simulink model "AC_base_1_VSM_2_22a"  (R2022a)
settings: Solver=ode3  StartTime=0.0  StopTime=8  FixedStep=HWSampleTime  RelTol=1e-3
undefined symbols (not defined in the file): ControlSampleTime, DiscIntNeverNeededParam, HWSampleTime, Ipwm_back, Ipwm_off, LCL, Manage, Oversample, Param, scaling_factor, SM, Ts, V_DC, VSMCTRL
libraries: fl_lib x100, nesl_utility x63, simulink x38, FriedrichLibrary x38, ee_lib x20, simulink_extras x14, TriphaseHardwaremodule x12, spsEdgeDetectorLib x2, StateMachines x2, slpidlib x2, spsPower3phInstantaneousLib x1
(part 2 of 7)

== system AC_base_1_VSM_2_22a/Variant Subsystem3/VSM/Inverter AverageMdl LC SimScape2/Modul F30 fixed DC voltage Average SimScape ==
  ctrl : Inport
  Bus Selector : BusSelector  OutputSignals=connect
  Phase Splitter : ee_lib/Connectors & References/Phase Splitter
  Rate Transition1 : RateTransition  Commented=on  Integrity=off  InitialCondition=-1  OutPortSampleTime=ControlSampleTime
  S_connect : ee_lib/Switches & Breakers/SPST Switch (Three-Phase)  R_closed=1e-9 Ohm  G_open=1e-6 1/Ohm  threshold=0.5 V  i_vT_specify=off  i_vT_priority=None  i_vT=0 A  i_vT_nominal_specify=off  i_vT_nominal_value=1  i_vT_nominal_unit=A  I_specify=off  I_priority=None  I=[ 0 0 0 ] A  I_nominal_specify=off  I_nominal_value=1  I_nominal_unit=A  V_specify=off  V_priority=None  V=[ 0 0 0 ] V  V_nominal_specify=off  V_nominal_value=1  V_nominal_unit=V  i_a_specify=off  i_a_priority=None  i_a=0 A  i_a_nominal_specify=off  i_a_nominal_value=1  i_a_nominal_unit=A  v_a_specify=off  v_a_priority=None  v_a=0 V  v_a_nominal_specify=off  v_a_nominal_value=1  v_a_nominal_unit=V  i_b_specify=off  i_b_priority=None  i_b=0 A  i_b_nominal_specify=off  i_b_nominal_value=1  i_b_nominal_unit=A  v_b_specify=off  v_b_priority=None  v_b=0 V  v_b_nominal_specify=off  v_b_nominal_value=1  v_b_nominal_unit=V  i_c_specify=off  i_c_priority=None  i_c=0 A  i_c_nominal_specify=off  i_c_nominal_value=1  i_c_nominal_unit=A  v_c_specify=off  v_c_priority=None  v_c=0 V  v_c_nominal_specify=off  v_c_nominal_value=1  v_c_nominal_unit=V
      settings: InternalSimscapePortConfiguration="{\"Bottom\":[],\"Left\":[{\"id\":\"vT\",\"label\":\"vT\",\"type\":\"input\"},{\"id\":\"N1\",\"label\":\"~1\",\"type\":\"foundation.electrical.three_phase\"}],\"Right\":[{\"id\":\"N2\",\"label\":\"~2\",\"type\":\"foundation.electrical.three_phase\"}],\"Top\":[]}"
  Simulink-PS Converter : nesl_utility/Simulink-PS Converter  PhysicalDomain=network_engine_domain  SubClassName=ps_input  LeftPortType=input  RightPortType=output  PseudoPeriodic=off  Frequencies=[]  NoiseDistribution=none  NoiseParameters=[]  Unit=1  AffineConversion=off  FilteringAndDerivatives=zero  SimscapeFilterOrder=1  InputFilterTimeConstant=0.001  UdotUserProvided=1
  ctrlSelect3 : Subsystem
  measMerge3 : Subsystem
  simscape_bridgefilter_aca : Subsystem  mask{L1=L1, R_L1=R_L1, C1=C1, R_C1=R_C1}
      mask prompts: L1 "Inductance L1 [H]"; R_L1 "Resistance of L1 [Ohm]"; C1 "Capacitance C1 [F]"; R_C1 "Parallel resistance of C1 [Ohm]"
      mask DialogControl LC Prompt: LC(L)(C)
      mask DialogControl GrpLC Prompt: LC(L)(C)-Filter
  simscape_bridgefilter_aca1 : Subsystem  mask{L1=L1, R_L1=R_L1, C1=C1, R_C1=R_C1}
      mask prompts: L1 "Inductance L1 [H]"; R_L1 "Resistance of L1 [Ohm]"; C1 "Capacitance C1 [F]"; R_C1 "Parallel resistance of C1 [Ohm]"
      mask DialogControl LC Prompt: LC(L)(C)
      mask DialogControl GrpLC Prompt: LC(L)(C)-Filter
  simscape_bridgefilter_aca2 : Subsystem  mask{L1=L1, R_L1=R_L1, C1=C1, R_C1=R_C1}
      mask prompts: L1 "Inductance L1 [H]"; R_L1 "Resistance of L1 [Ohm]"; C1 "Capacitance C1 [F]"; R_C1 "Parallel resistance of C1 [Ohm]"
      mask DialogControl LC Prompt: LC(L)(C)
      mask DialogControl GrpLC Prompt: LC(L)(C)-Filter
  N : PMIOPort  Side=Left
  ABC : PMIOPort  Port=2  Side=Right
  meas : Outport  VectorParamsAs1DForOutWhenUnconnected=off
  measf : Outport  Port=2  VectorParamsAs1DForOutWhenUnconnected=off
  wires:
  ctrlSelect3/1(ctrl1) -> Bus Selector/1, simscape_bridgefilter_aca/1(ctrl)
  [ctrl3] -> simscape_bridgefilter_aca2/1(ctrl)
  [ctrl2] -> simscape_bridgefilter_aca1/1(ctrl)
  ctrlSelect3/2(ctrl2) -> [ctrl2]
  ctrlSelect3/3(ctrl3) -> [ctrl3]
  ctrl/1 -> ctrlSelect3/1(ctrl)
  [meas2] -> measMerge3/2(meas2)
  simscape_bridgefilter_aca2/1(meas) -> [meas3]
  simscape_bridgefilter_aca1/1(meas) -> [meas2]
  [meas3] -> measMerge3/3(meas3)
  simscape_bridgefilter_aca/1(meas) -> measMerge3/1(meas1)
  measMerge3/1(meas) -> meas/1, measf/1
  Bus Selector/1 -> [connect]  "<connect>"
  [connect] -> Simulink-PS Converter/1
  connections:
  simscape_bridgefilter_aca/LConn2 -- simscape_bridgefilter_aca1/LConn2 -- simscape_bridgefilter_aca2/LConn2 -- N/RConn1
  simscape_bridgefilter_aca/RConn1 -- simscape_bridgefilter_aca2/RConn1 -- simscape_bridgefilter_aca1/RConn1
  simscape_bridgefilter_aca2/LConn1 -- Phase Splitter/RConn3
  Phase Splitter/RConn1 -- simscape_bridgefilter_aca/LConn1
  simscape_bridgefilter_aca1/LConn1 -- Phase Splitter/RConn2
  Simulink-PS Converter/RConn1 -- S_connect/LConn1
  S_connect/LConn2 -- ABC/RConn1
  S_connect/RConn1 -- Phase Splitter/LConn1

== system AC_base_1_VSM_2_22a/Variant Subsystem3/VSM/VSM1/MeasInv1 ==
  SimOut : Inport
  Bus Selector1 : BusSelector  OutputSignals=meas_u_dc,meas_u_cap,meas_u_out,meas_i_inverter,meas_i_out,connection_state,enabled
  Meas_Inv1 : Scope  NumInputPorts=7
  To Workspace1 : ToWorkspace  VariableName=MeasAC_Ucap  SampleTime=-1
  To Workspace2 : ToWorkspace  VariableName=MeasAC_Uout  SampleTime=-1
  To Workspace3 : ToWorkspace  VariableName=MeasAC_Iinv  SampleTime=-1
  To Workspace4 : ToWorkspace  VariableName=MeasAC_Iout  SampleTime=-1
  To Workspace7 : ToWorkspace  VariableName=MeasAC_Udc  SampleTime=-1
  wires:
  Bus Selector1/7 -> Meas_Inv1/7  "<enabled>"
  Bus Selector1/6 -> Meas_Inv1/6  "<connection_state>"
  Bus Selector1/5 -> To Workspace4/1, Meas_Inv1/5  "<meas_i_out>"
  Bus Selector1/4 -> To Workspace3/1, Meas_Inv1/4  "<meas_i_inverter>"
  Bus Selector1/3 -> To Workspace2/1, Meas_Inv1/3  "<meas_u_out>"
  Bus Selector1/2 -> To Workspace1/1, Meas_Inv1/2  "<meas_u_cap>"
  Bus Selector1/1 -> To Workspace7/1, Meas_Inv1/1  "<meas_u_dc>"
  SimOut/1 -> Bus Selector1/1

== system AC_base_1_VSM_2_22a/Variant Subsystem3/VSM/VSM1/VSM ==
  cmd : Inport
  meas : Inport  Port=2
  BUS_GENERATION : Subsystem
  CONTROL : Subsystem
  MANAGEMENT : Subsystem  mask(VSMCC Management){Mgn=Ctrl.Mgn}
      mask prompts: Mgn "Mgn Parameters"
      mask help:
      | Mgn(.PQSpRateUp, .PQSpRateDown, PQSpMax, .PQSpMin)
      |
      | Parameter nicht auf der Maske:
      | ControlSampleTime
  Meas : Subsystem  mask(Messeinrichtung für VSM mit CC){PU=pu, PLL=Ctrl.PLL}
      mask prompts: PU "PU System"; PLL "PLL Parameters"
      mask help:
      | PU System(.Vb, .Ib)
      |
      | PLL Parameter (.kp, .ki)
      |
      | Parameter nicht auf der Maske:
      | NrChannels
      | ControlSampleTime
  ctrl : Outport  VectorParamsAs1DForOutWhenUnconnected=off  LockScale=on
  feedback : Outport  Port=2  VectorParamsAs1DForOutWhenUnconnected=off
  diag : Outport  Port=3  VectorParamsAs1DForOutWhenUnconnected=off
  wires:
  meas/1 -> Meas/1(MEASIN)
  cmd/1 -> MANAGEMENT/1(CMD)
  CONTROL/1(CONTROL) -> Meas/2("CONTROL "), BUS_GENERATION/2(CONTROL)
  BUS_GENERATION/1(ctrl) -> ctrl/1
  BUS_GENERATION/2(feedback) -> feedback/1
  CONTROL/2(diagCtrl) -> diag/1
  MANAGEMENT/1(MANAGE) -> CONTROL/1(MANAGE), BUS_GENERATION/1(MANAGE)
  Meas/1(MEAS) -> CONTROL/2(MEAS), MANAGEMENT/2(MEAS)

== system AC_base_1_VSM_2_22a/Variant Subsystem3/VSM/VSM1/command_center ==
  note: State Machine for TP <-> WP SIM
      |
      | State Index:
      | 0: Error
      | 1: Stop
      | 2: Ready (Precharge, Connected + Enable DC)
      | 3: Connect AC
      | 4: Enable AC
  Feed_AC : Inport
  Feed_DC : Inport  Port=2
  Bus Assignment : BusAssignment  AssignedSignals=Manage.connect,Manage.enable,Param.VSM.sp_PQ,Param.VSM.sp_E
  Bus Selector2 : BusSelector  OutputSignals=connect,enable
  Bus Creator1 : BusCreator  Inputs=2
  Constant : Constant
  Display1 : Display
  Display2 : Display
  Display5 : Display
  Error ACK : Subsystem
      settings: OpenFcn=|
      | switch get_param([gcb '/Toggle'],'Value')
      |     case '1'
      |         set_param([gcb '/Toggle'],'Value', '0');
      |         set_param(gcb,'BackgroundColor','[0.8500    0.3250    0.0980]');
      |     case '0'
      |         set_param([gcb '/Toggle'],'Value', '1');
      |         set_param(gcb,'BackgroundColor','[0.4660    0.6740    0.1880]');
      | end
      mask Display: port_label('output',1,'')
  Rate Transition3 : RateTransition  Integrity=off  OutPortSampleTime=ControlSampleTime
  Shortcut1 : Subsystem  mask{path=./ControlLibrary/FriedrichLibrary.slx}
      settings: OpenFcn=findsimscopes
      mask Display: disp('Open Scopes...')
  Step3 : Step  Time=5.0+100  Before=[0.5 0]*-1  After=[0.1 0]  SampleTime=0
  Step4 : Step  Time=0  SampleTime=0
  Subsystem : Subsystem
  cmd_VSM : Subsystem  AncestorBlock=ControLibrary/cmd_VSM template
  cmd_tp : Outport  VectorParamsAs1DForOutWhenUnconnected=off
  cmd_ac : Outport  Port=2  VectorParamsAs1DForOutWhenUnconnected=off
  wires:
  Rate Transition3/1 -> cmd_ac/1
  cmd_VSM/1(cmd_ac) -> Bus Assignment/1
  Bus Assignment/1 -> Rate Transition3/1
  Error ACK/1(Out) -> Bus Creator1/1  "error_ack"
  Bus Creator1/1 -> cmd_tp/1
  Bus Selector2/1 -> Display1/1, Bus Assignment/2  "<connect>"
  Bus Selector2/2 -> Display2/1, Bus Assignment/3  "<enable>"
  Subsystem/1(precharge) -> Bus Creator1/2, Display5/1
  Feed_AC/1 -> Subsystem/1(In1)
  Feed_DC/1 -> Subsystem/2(In2)
  Subsystem/2(cmd_ac) -> Bus Selector2/1
  Step4/1 -> Subsystem/Enable
  Step3/1 -> Bus Assignment/4
  Constant/1 -> Bus Assignment/5

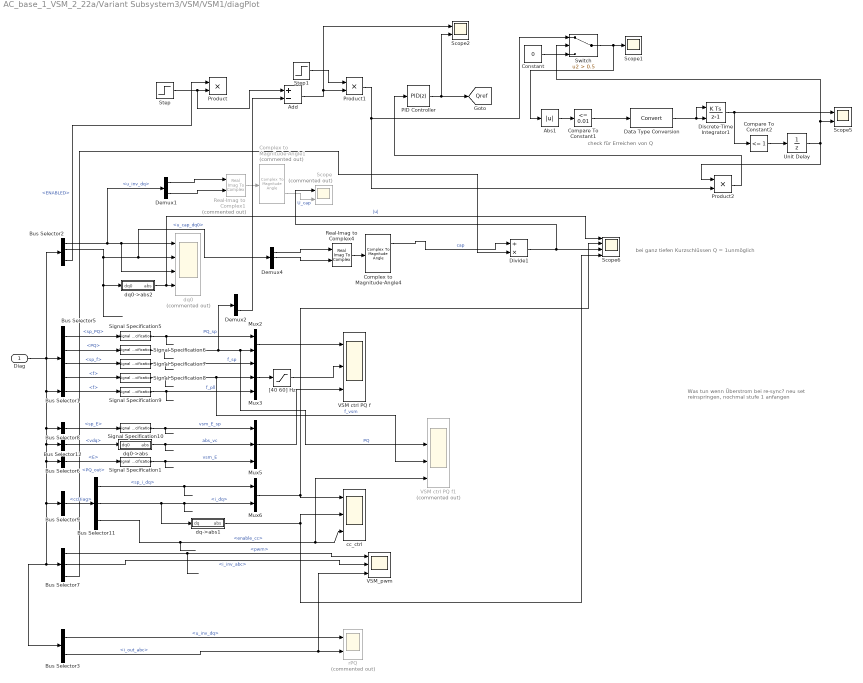
== system AC_base_1_VSM_2_22a/Variant Subsystem3/VSM/VSM1/diagPlot ==
  note: Was tun wenn Überstrom bei re-sync?
      |
      | neu set reinspringen, nochmal stufe 1 anfangen
  note: bei ganz tiefen Kurzschlüssen Q = 1unmöglich
  note: check für Erreichen von Q
  Diag : Inport
  Abs1 : Abs  SaturateOnIntegerOverflow=off
  Add : Sum  Inputs=+-
  Bus Selector1 : BusSelector  OutputSignals=measDiag.PLL.f
  Bus Selector11 : BusSelector  OutputSignals=sp_i_dq,i_dq,enable_cc
  Bus Selector12 : BusSelector  OutputSignals=measDiag.PLL.vdq
  Bus Selector2 : BusSelector  OutputSignals=u_inv_dq,measDiag.u_cap.u_cap_dq0,measDiag.u_cap.u_cap_abc,manage.ENABLED
  Bus Selector3 : BusSelector  OutputSignals=u_inv_dq,measDiag.i_out.i_out_abc
  Bus Selector5 : BusSelector  OutputSignals=manage.sp_VSM.sp_PQ,measDiag.PQ,manage.sp_VSM.sp_f,vsmDiag.f
  Bus Selector6 : BusSelector  OutputSignals=vsmDiag.E
  Bus Selector7 : BusSelector  OutputSignals=pwmDiag.pwm,measDiag.i_inv.i_inv_abc,measDiag.PQ_out
  Bus Selector8 : BusSelector  OutputSignals=vsmDiag.sp_VSM.sp_E
  Bus Selector9 : BusSelector  OutputSignals=ccDiag
  Compare To Constant1 : simulink/Logic and Bit Operations/Compare To Constant  relop=<=  const=0.01  OutDataTypeStr=boolean
  Compare To Constant2 : simulink/Logic and Bit Operations/Compare To Constant  relop=<=  const=1  OutDataTypeStr=boolean
  Complex to Magnitude-Angle1 : ComplexToMagnitudeAngle  Commented=on
  Complex to Magnitude-Angle4 : ComplexToMagnitudeAngle
  Constant : Constant  Value=0
  Data Type Conversion : DataTypeConversion  SaturateOnIntegerOverflow=off  RndMeth=Floor
  Demux1 : Demux  Outputs=2
  Demux2 : Demux  Outputs=2
  Demux4 : Demux  Outputs=3
  Discrete-Time Integrator1 : DiscreteIntegrator  ExternalReset=rising  SampleTime=-1  ICPrevOutput=DiscIntNeverNeededParam  ICPrevScaledInput=DiscIntNeverNeededParam
  Divide1 : Product  Inputs=/*
  Mux2 : Mux  Inputs=2
  Mux3 : Mux  Inputs=3
  Mux5 : Mux  Inputs=3
  Mux6 : Mux  Inputs=2
  PID Controller : slpidlib/PID Controller  Controller=PID  Form=Parallel  TimeDomain=Discrete-time  UseExternalTs=off  SampleTime=-1  IntegratorMethod=Forward Euler  FilterMethod=Forward Euler  ControllerParametersSource=internal  P=0.1  I=1  UseKiTs=off  D=0  N=100  UseFilter=on  TunerSelectOption=Transfer Function Based (PID Tuner App)  InitialConditionSource=internal  InitialConditionForIntegrator=1  InitialConditionForFilter=0  DifferentiatorICPrevScaledInput=0  ExternalReset=none  TrackingMode=off  Kt=1  LimitOutput=off  SatLimitsSource=internal  UpperSaturationLimit=inf  LowerSaturationLimit=-inf  LinearizeAsGain=on  AntiWindupMode=none  Kb=1  POutMin=[]  POutMax=[]  IOutMin=[]  IOutMax=[]  DOutMin=[]  DOutMax=[]  NOutMin=[]  NOutMax=[]  SumOutMin=[]  SumOutMax=[]  SaturationOutMin=[]  SaturationOutMax=[]  PParamMin=[]  PParamMax=[]  IParamMin=[]  IParamMax=[]  DParamMin=[]  DParamMax=[]  NParamMin=[]  NParamMax=[]  KbParamMin=[]  KbParamMax=[]  KtParamMin=[]  KtParamMax=[]  KbOutMin=[]  KbOutMax=[]  KtOutMin=[]  KtOutMax=[]  IntegratorOutMin=[]  IntegratorOutMax=[]  FilterOutMin=[]  FilterOutMax=[]  SumI1OutMin=[]  SumI1OutMax=[]  SumI2OutMin=[]  SumI2OutMax=[]  SumI3OutMin=[]  SumI3OutMax=[]  SumI4OutMin=[]  SumI4OutMax=[]  SumDOutMin=[]  SumDOutMax=[]  DifferentiatorOutMin=[]  DifferentiatorOutMax=[]  FilterDiffOutCoefMin=[]  FilterDiffOutCoefMax=[]  ReciprocalOutMin=[]  ReciprocalOutMax=[]  SumDenOutMin=[]  SumDenOutMax=[]  SumNumOutMin=[]  SumNumOutMax=[]  DivideOutMin=[]  DivideOutMax=[]  UdiffTsProdOutMin=[]  UdiffTsProdOutMax=[]  NTsProdOutMin=[]  NTsProdOutMax=[]  UintegralTsProdOutMin=[]  UintegralTsProdOutMax=[]  UngainTsProdOutMin=[]  UngainTsProdOutMax=[]  IntegratorContinuousStateAttributes=''  IntegratorStateMustResolveToSignalObject=off  IntegratorRTWStateStorageClass=Auto  FilterContinuousStateAttributes=''  FilterStateMustResolveToSignalObject=off  FilterRTWStateStorageClass=Auto  ParallelPVariant=InternalParameters  IdealPVariant=Disabled  IVariant=InternalParameters  DVariant=InternalParameters  IntegratorVariant=Discrete  SatVariant=Disabled  AWVariant=Passthrough  PCopyVariant=Disabled  TRVariant=Disabled  FdbkBlocksVariant=Forward  IdealPFdbkVariant=Disabled  SatFdbkVariant=Disabled  DerivativeFilterVariant=ForwardEulerFilter  NVariant=InternalParameters  NCopyVariant=Disabled  FilterICVariant=InternalICsFilter  IntegratorICVariant=InternalICs  ExternalResetVariant=Disabled  TRSumVariant=Passthrough  SumFdbkVariant=Disabled  SumVariant=Sum_PID  TsampFilterVariant=InternalTs  TsampNgainVariant=Passthrough  TsampIntegralVariant=Disabled_SignalSpec  ExternalSaturationOutDataTypeStr=Inherit: Same as second input
  Product : Product
  Product1 : Product
  Product2 : Product
  Real-Imag to Complex1 : RealImagToComplex  Commented=on
  Real-Imag to Complex4 : RealImagToComplex
  Scope : Scope  Commented=on  NumInputPorts=2
  Scope1 : Scope
  Scope2 : Scope  NumInputPorts=2
  Scope5 : Scope  NumInputPorts=2
  Scope6 : Scope  NumInputPorts=4
  Signal Specification{1,5..10} (7 alike) : SignalSpecification
  Step : Step  Time=6+20  Before=0.2  After=0.1  SampleTime=0
  Step1 : Step  Time=4.5  Before=1  SampleTime=0
  Switch : Switch  Criteria=u2 > Threshold  Threshold=0.5  SaturateOnIntegerOverflow=off  InputSameDT=off
  Unit Delay : UnitDelay  InitialCondition=1  SampleTime=-1  HasFrameUpgradeWarning=on
  VSM ctrl PQ f : Scope  NumInputPorts=3
  VSM ctrl PQ f1 : Scope  Commented=on  NumInputPorts=4
  VSM_pwm : Scope  NumInputPorts=3
  "[40 60] Hz" : Saturate  UpperLimit=60  LowerLimit=40
  cc_ctrl : Scope  NumInputPorts=3
  dq->abs1 : Subsystem
  dq0 : Scope  Commented=on  NumInputPorts=4
  dq0->abs : Subsystem
  dq0->abs2 : Subsystem
  rPQ : Scope  Commented=on  NumInputPorts=2
  tag scope: Qref=global
  wires:
  Diag/1 -> Bus Selector2/1, Bus Selector6/1, Bus Selector7/1, Bus Selector3/1, Bus Selector9/1, Bus Selector12/1, Bus Selector8/1, Bus Selector1/1, Bus Selector5/1
  Bus Selector7/1 -> VSM_pwm/1  "<pwm>"
  Mux5/1 -> VSM ctrl PQ f/3
  dq0->abs/1(abs) -> Mux5/2  "abs_vc"
  Bus Selector8/1 -> Signal Specification10/1  "<sp_E>"
  Bus Selector11/1 -> Mux6/1  "<sp_i_dq>"
  Bus Selector9/1 -> Bus Selector11/1  "<ccDiag>"
  Bus Selector12/1 -> dq0->abs/1(dq0)  "<vdq>"
  Bus Selector11/3 -> VSM ctrl PQ f1/4, cc_ctrl/3  "<enable_cc>"
  Mux6/1 -> Scope6/2, cc_ctrl/1
  Bus Selector5/1 -> Signal Specification5/1  "<sp_PQ>"
  Bus Selector5/2 -> Signal Specification6/1  "<PQ>"
  Bus Selector5/3 -> Signal Specification7/1  "<sp_f>"
  Bus Selector5/4 -> Signal Specification8/1  "<f>"
  Signal Specification5/1 -> Mux2/1  "PQ_sp"
  Signal Specification7/1 -> Mux3/1  "f_sp"
  Signal Specification8/1 -> VSM ctrl PQ f1/3, Mux3/2  "f_vsm"
  Mux2/1 -> VSM ctrl PQ f/1
  Mux3/1 -> "[40 60] Hz"/1
  Bus Selector1/1 -> Signal Specification9/1  "<f>"
  Signal Specification9/1 -> Mux3/3  "f_pll"
  Signal Specification10/1 -> Mux5/1  "vsm_E_sp"
  Bus Selector11/2 -> dq->abs1/1(dq), Mux6/2  "<i_dq>"
  dq->abs1/1(abs) -> cc_ctrl/2, Scope6/4
  Bus Selector6/1 -> Signal Specification1/1  "<E>"
  Signal Specification1/1 -> Mux5/3  "vsm_E"
  "[40 60] Hz"/1 -> VSM ctrl PQ f/2
  dq0->abs2/1(abs) -> Scope6/1, dq0/4  "|u|"
  Bus Selector3/2 -> VSM_pwm/3, rPQ/2  "<i_out_abc>"
  Bus Selector3/1 -> rPQ/1  "<u_inv_dq>"
  Bus Selector7/2 -> VSM_pwm/2  "<i_inv_abc>"
  Bus Selector2/2 -> dq0->abs2/1(dq0), Demux4/1, dq0/2  "<u_cap_dq0>"
  Real-Imag to Complex4/1 -> Complex to Magnitude-Angle4/1
  Demux4/1 -> Real-Imag to Complex4/1
  Demux4/2 -> Real-Imag to Complex4/2
  Complex to Magnitude-Angle4/1 -> Divide1/1  "cap"
  Signal Specification6/1 -> Demux2/1, VSM ctrl PQ f1/2, Mux2/2  "PQ"
  Bus Selector7/3 -> Divide1/2  "<PQ_out>"
  Demux1/2 -> Real-Imag to Complex1/2
  Demux1/1 -> Real-Imag to Complex1/1
  Real-Imag to Complex1/1 -> Complex to Magnitude-Angle1/1
  Complex to Magnitude-Angle1/2 -> Scope/2  "U_cap"
  Bus Selector2/1 -> Demux1/1, dq0/3, dq0/1  "<u_inv_dq>"
  Demux2/2 -> Add/2
  PID Controller/1 -> [Qref], Scope2/2
  Step/1 -> Add/1, Product/2
  Bus Selector2/4 -> Product/1  "<ENABLED>"
  Add/1 -> Scope2/1, Product1/2
  Product1/1 -> Product2/2, Switch/1
  Step1/1 -> Product1/1
  Abs1/1 -> Compare To Constant1/1
  Compare To Constant1/1 -> Data Type Conversion/1
  Discrete-Time Integrator1/1 -> Scope5/1, Compare To Constant2/1
  Data Type Conversion/1 -> Discrete-Time Integrator1/2, Discrete-Time Integrator1/1
  Compare To Constant2/1 -> Unit Delay/1
  Product2/1 -> PID Controller/1
  Unit Delay/1 -> Switch/2, Scope5/2, Product2/1
  Constant/1 -> Switch/3
  Switch/1 -> Abs1/1, Scope1/1
  Divide1/1 -> Scope/1, Scope6/3

== system AC_base_1_VSM_2_22a/Variant Subsystem1/VSM/Inverter AverageMdl LC SimScape2/Modul F30 fixed DC voltage Average SimScape/ctrlSelect3 ==
  ctrl : Inport
  Bus Creator1 : BusCreator  Inputs=3
  Bus Creator2 : BusCreator  Inputs=3
  Bus Creator3 : BusCreator  Inputs=3
  Bus Selector : BusSelector  OutputSignals=pwm,connect,enable
  Compare To Constant : simulink/Logic and Bit Operations/Compare To Constant  relop=<  const=0.5  OutDataTypeStr=boolean
  Constant : Constant
  Data Type Conversion : DataTypeConversion  OutDataTypeStr=double  SaturateOnIntegerOverflow=off  RndMeth=Floor
  Data Type Conversion1 : DataTypeConversion  OutDataTypeStr=double  SaturateOnIntegerOverflow=off  RndMeth=Floor
  Rate Transition : RateTransition  Integrity=off  Deterministic=off  OutPortSampleTime=0
  Selector1 : Selector  InputPortWidth=3  IndexOptions=Index vector (dialog)  Indices=[1]  OutputSizes=1
  Selector2 : Selector  InputPortWidth=3  IndexOptions=Index vector (dialog)  Indices=2  OutputSizes=1
  Selector3 : Selector  InputPortWidth=3  IndexOptions=Index vector (dialog)  Indices=3  OutputSizes=1
  Sum of Elements : Sum  Inputs=+
  Sum of Elements1 : Sum  Inputs=+  SampleTime=ControlSampleTime
  ctrl1 : Outport  VectorParamsAs1DForOutWhenUnconnected=off
  ctrl2 : Outport  Port=2  VectorParamsAs1DForOutWhenUnconnected=off
  ctrl3 : Outport  Port=3  VectorParamsAs1DForOutWhenUnconnected=off
  wires:
  Compare To Constant/1 -> Data Type Conversion/1
  Bus Selector/3 -> Compare To Constant/1  "<enable>"
  Bus Selector/2 -> Data Type Conversion1/1  "<connect>"
  Constant/1 -> Sum of Elements1/1, Sum of Elements/1
  Data Type Conversion1/1 -> Bus Creator1/2, Bus Creator3/2, Bus Creator2/2  "connect"
  Data Type Conversion/1 -> Bus Creator3/3, Bus Creator2/3, Bus Creator1/3  "enable"
  Bus Selector/1 -> Rate Transition/1  "<pwm>"
  Selector3/1 -> Bus Creator2/1  "pwm"
  Bus Creator2/1 -> ctrl3/1
  ctrl/1 -> Bus Selector/1
  Bus Creator1/1 -> ctrl1/1
  Selector2/1 -> Bus Creator3/1  "pwm"
  Bus Creator3/1 -> ctrl2/1
  Selector1/1 -> Bus Creator1/1  "pwm"
  Rate Transition/1 -> Selector2/1, Selector3/1, Selector1/1

== system AC_base_1_VSM_2_22a/Variant Subsystem1/VSM/Inverter AverageMdl LC SimScape2/Modul F30 fixed DC voltage Average SimScape/measMerge3 ==
  meas1 : Inport
  meas2 : Inport  Port=2
  meas3 : Inport  Port=3
  measMerge123 : Subsystem
  meas : Outport  VectorParamsAs1DForOutWhenUnconnected=off
  wires:
  meas1/1 -> measMerge123/1(meas1)
  measMerge123/1(meas) -> meas/1
  meas2/1 -> measMerge123/2(meas2)
  meas3/1 -> measMerge123/3(meas3)

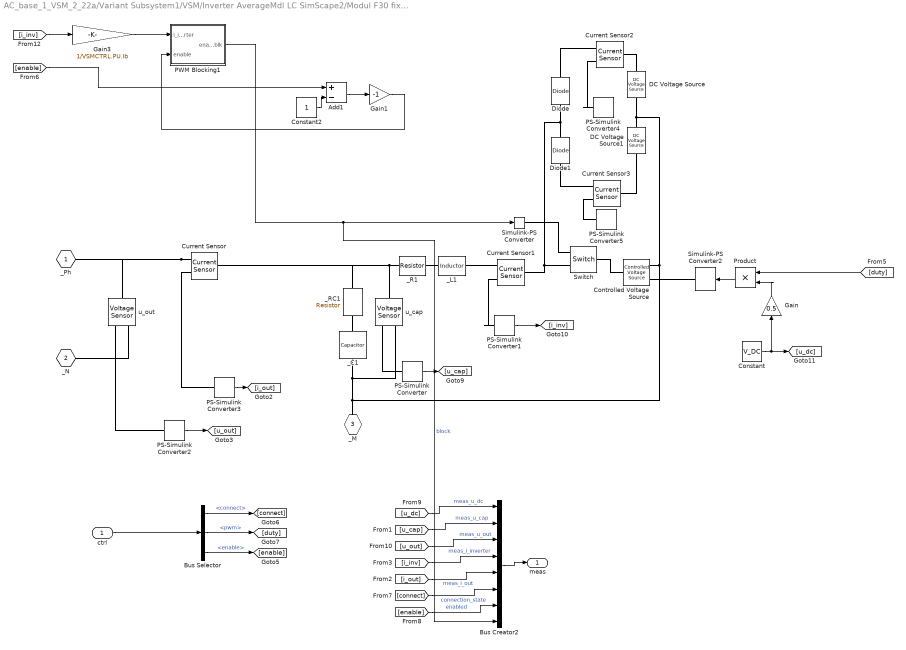
== system AC_base_1_VSM_2_22a/Variant Subsystem1/VSM/Inverter AverageMdl LC SimScape2/Modul F30 fixed DC voltage Average SimScape/simscape_bridgefilter_aca ==
  ctrl : Inport
  Add1 : Sum  Inputs=+-
  Bus Creator2 : BusCreator  Inputs=8
  Bus Selector : BusSelector  OutputSignals=connect,pwm,enable
  Constant : Constant  Value=V_DC
  Constant2 : Constant
  Controlled Voltage Source : fl_lib/Electrical/Electrical Sources/Controlled Voltage Source
  Current Sensor{,1..3} (4 alike) : fl_lib/Electrical/Electrical Sensors/Current Sensor
  DC Voltage Source : fl_lib/Electrical/Electrical Sources/DC Voltage Source  v0=V_DC/2 V
  DC Voltage Source1 : fl_lib/Electrical/Electrical Sources/DC Voltage Source  v0=V_DC/2 V
  Diode : fl_lib/Electrical/Electrical Elements/Diode  Vf=0.6 V  Ron=0.001*scaling_factor Ohm  Goff=1e-8 1/Ohm  i_specify=off  i_priority=None  i=0 A  i_nominal_specify=off  i_nominal_value=1  i_nominal_unit=A  v_specify=off  v_priority=None  v=0 V  v_nominal_specify=off  v_nominal_value=1  v_nominal_unit=V
  Diode1 : fl_lib/Electrical/Electrical Elements/Diode  Vf=0.6 V  Ron=0.001*scaling_factor Ohm  Goff=1e-8 1/Ohm  i_specify=off  i_priority=None  i=0 A  i_nominal_specify=off  i_nominal_value=1  i_nominal_unit=A  v_specify=off  v_priority=None  v=0 V  v_nominal_specify=off  v_nominal_value=1  v_nominal_unit=V
  Gain : Gain  Gain=0.5
  Gain1 : Gain  Gain=-1
  Gain3 : Gain  Gain=1/VSMCTRL.PU.Ib
  PS-Simulink Converter{,1..5} (6 alike) : nesl_utility/PS-Simulink Converter  PhysicalDomain=network_engine_domain  SubClassName=ps_output  LeftPortType=input  RightPortType=output  PseudoPeriodic=off  Frequencies=[]  VectorFormat=1-D array  Unit=1  AffineConversion=off
  PWM Blocking1 : Subsystem
  Product : Product
  Simulink-PS Converter : nesl_utility/Simulink-PS Converter  PhysicalDomain=network_engine_domain  SubClassName=ps_input  LeftPortType=input  RightPortType=output  PseudoPeriodic=off  Frequencies=[]  NoiseDistribution=none  NoiseParameters=[]  Unit=1  AffineConversion=off  FilteringAndDerivatives=provide  SimscapeFilterOrder=1  InputFilterTimeConstant=0.001  UdotUserProvided=0
  Simulink-PS Converter2 : nesl_utility/Simulink-PS Converter  PhysicalDomain=network_engine_domain  SubClassName=ps_input  LeftPortType=input  RightPortType=output  PseudoPeriodic=off  Frequencies=[]  NoiseDistribution=none  NoiseParameters=[]  Unit=1  AffineConversion=off  FilteringAndDerivatives=zero  SimscapeFilterOrder=1  InputFilterTimeConstant=0.001  UdotUserProvided=1
  Switch : fl_lib/Electrical/Electrical Elements/Switch  R_closed=0.001*scaling_factor Ohm  G_open=1e-8 1/Ohm  Threshold=0.5  i_specify=off  i_priority=None  i=0 A  i_nominal_specify=off  i_nominal_value=1  i_nominal_unit=A  v_specify=off  v_priority=None  v=0 V  v_nominal_specify=off  v_nominal_value=1  v_nominal_unit=V
  _C1 : fl_lib/Electrical/Electrical Elements/Capacitor  c=C1 F  r=1e-6 Ohm  g=0 1/Ohm  i_specify=off  i_priority=None  i=0 A  i_nominal_specify=off  i_nominal_value=1  i_nominal_unit=A  v_specify=off  v_priority=None  v=0 V  v_nominal_specify=off  v_nominal_value=1  v_nominal_unit=V  vc_specify=off  vc_priority=None  vc=0 V  vc_nominal_specify=off  vc_nominal_value=1  vc_nominal_unit=V
  _L1 : fl_lib/Electrical/Electrical Elements/Inductor  l=L1 H  r=0 Ohm  g=1e-9 1/Ohm  i_specify=off  i_priority=None  i=0 A  i_nominal_specify=off  i_nominal_value=1  i_nominal_unit=A  v_specify=off  v_priority=None  v=0 V  v_nominal_specify=off  v_nominal_value=1  v_nominal_unit=V  i_L_specify=off  i_L_priority=None  i_L=0 A  i_L_nominal_specify=off  i_L_nominal_value=1  i_L_nominal_unit=A
  _R1 : fl_lib/Electrical/Electrical Elements/Resistor  R=R_L1 Ohm  i_specify=off  i_priority=None  i=0 A  i_nominal_specify=off  i_nominal_value=1  i_nominal_unit=A  v_specify=off  v_priority=None  v=0 V  v_nominal_specify=off  v_nominal_value=1  v_nominal_unit=V
  _RC1 : fl_lib/Electrical/Electrical Elements/Resistor  R=R_C1 Ohm  i_specify=off  i_priority=None  i=0 A  i_nominal_specify=off  i_nominal_value=1  i_nominal_unit=A  v_specify=off  v_priority=None  v=0 V  v_nominal_specify=off  v_nominal_value=1  v_nominal_unit=V
  u_cap : fl_lib/Electrical/Electrical Sensors/Voltage Sensor
  u_out : fl_lib/Electrical/Electrical Sensors/Voltage Sensor
  _Ph : PMIOPort  Side=Left
  _N : PMIOPort  Port=2  Side=Left
  _M : PMIOPort  Port=3  Side=Right
  meas : Outport  VectorParamsAs1DForOutWhenUnconnected=off
  wires:
  Gain1/1 -> PWM Blocking1/2(enable)
  [enable] -> Add1/1
  PWM Blocking1/1(enable_blk) -> Simulink-PS Converter/1, Bus Creator2/8  "block"
  [i_inv] -> Gain3/1
  Gain3/1 -> PWM Blocking1/1(i_inverter)
  Add1/1 -> Gain1/1
  Constant2/1 -> Add1/2
  PS-Simulink Converter3/1 -> [i_out]
  Gain/1 -> Product/2
  [duty] -> Product/1
  Constant/1 -> Gain/1, [u_dc]
  Product/1 -> Simulink-PS Converter2/1
  PS-Simulink Converter2/1 -> [u_out]
  PS-Simulink Converter1/1 -> [i_inv]
  PS-Simulink Converter/1 -> [u_cap]
  [u_dc] -> Bus Creator2/1  "meas_u_dc"
  Bus Creator2/1 -> meas/1
  [enable] -> Bus Creator2/7  "enabled"
  Bus Selector/3 -> [enable]  "<enable>"
  [u_cap] -> Bus Creator2/2  "meas_u_cap"
  [u_out] -> Bus Creator2/3  "meas_u_out"
  [i_inv] -> Bus Creator2/4  "meas_i_inverter"
  [i_out] -> Bus Creator2/5  "meas_i_out"
  ctrl/1 -> Bus Selector/1
  [connect] -> Bus Creator2/6  "connection_state"
  Bus Selector/1 -> [connect]  "<connect>"
  Bus Selector/2 -> [duty]  "<pwm>"
  connections:
  Current Sensor2/LConn1 -- DC Voltage Source/LConn1
  PS-Simulink Converter5/LConn1 -- Current Sensor3/RConn1
  Current Sensor2/RConn2 -- Diode/RConn1
  PS-Simulink Converter4/LConn1 -- Current Sensor2/RConn1
  Current Sensor3/RConn2 -- Diode1/LConn1
  Current Sensor3/LConn1 -- DC Voltage Source1/RConn1
  Simulink-PS Converter/RConn1 -- Switch/RConn1
  Controlled Voltage Source/LConn1 -- Switch/LConn1
  Diode/LConn1 -- Switch/RConn2 -- Current Sensor1/LConn1 -- Diode1/RConn1
  _RC1/RConn1 -- _C1/LConn1
  PS-Simulink Converter3/LConn1 -- Current Sensor/RConn1
  PS-Simulink Converter2/LConn1 -- u_out/RConn1
  PS-Simulink Converter1/LConn1 -- Current Sensor1/RConn1
  PS-Simulink Converter/LConn1 -- u_cap/RConn1
  Simulink-PS Converter2/RConn1 -- Controlled Voltage Source/RConn1
  u_out/RConn2 -- _N/RConn1
  Current Sensor/RConn2 -- _Ph/RConn1 -- u_out/LConn1
  DC Voltage Source1/LConn1 -- Controlled Voltage Source/RConn2 -- _C1/RConn1 -- u_cap/RConn2 -- _M/RConn1 -- DC Voltage Source/RConn1
  _R1/LConn1 -- u_cap/LConn1 -- Current Sensor/LConn1 -- _RC1/LConn1
  Current Sensor1/RConn2 -- _L1/RConn1
  _R1/RConn1 -- _L1/LConn1

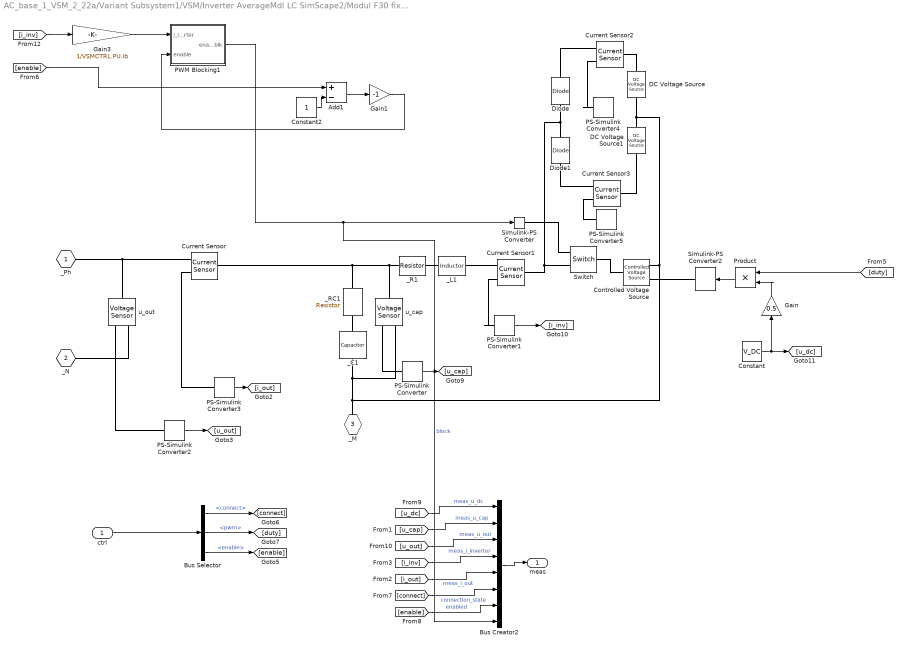
== system AC_base_1_VSM_2_22a/Variant Subsystem1/VSM/Inverter AverageMdl LC SimScape2/Modul F30 fixed DC voltage Average SimScape/simscape_bridgefilter_aca1 ==
  ctrl : Inport
  Add1 : Sum  Inputs=+-
  Bus Creator2 : BusCreator  Inputs=8
  Bus Selector : BusSelector  OutputSignals=connect,pwm,enable
  Constant : Constant  Value=V_DC
  Constant2 : Constant
  Controlled Voltage Source : fl_lib/Electrical/Electrical Sources/Controlled Voltage Source
  Current Sensor{,1..3} (4 alike) : fl_lib/Electrical/Electrical Sensors/Current Sensor
  DC Voltage Source : fl_lib/Electrical/Electrical Sources/DC Voltage Source  v0=V_DC/2 V
  DC Voltage Source1 : fl_lib/Electrical/Electrical Sources/DC Voltage Source  v0=V_DC/2 V
  Diode : fl_lib/Electrical/Electrical Elements/Diode  Vf=0.6 V  Ron=0.001*scaling_factor Ohm  Goff=1e-8 1/Ohm  i_specify=off  i_priority=None  i=0 A  i_nominal_specify=off  i_nominal_value=1  i_nominal_unit=A  v_specify=off  v_priority=None  v=0 V  v_nominal_specify=off  v_nominal_value=1  v_nominal_unit=V
  Diode1 : fl_lib/Electrical/Electrical Elements/Diode  Vf=0.6 V  Ron=0.001*scaling_factor Ohm  Goff=1e-8 1/Ohm  i_specify=off  i_priority=None  i=0 A  i_nominal_specify=off  i_nominal_value=1  i_nominal_unit=A  v_specify=off  v_priority=None  v=0 V  v_nominal_specify=off  v_nominal_value=1  v_nominal_unit=V
  Gain : Gain  Gain=0.5
  Gain1 : Gain  Gain=-1
  Gain3 : Gain  Gain=1/VSMCTRL.PU.Ib
  PS-Simulink Converter{,1..5} (6 alike) : nesl_utility/PS-Simulink Converter  PhysicalDomain=network_engine_domain  SubClassName=ps_output  LeftPortType=input  RightPortType=output  PseudoPeriodic=off  Frequencies=[]  VectorFormat=1-D array  Unit=1  AffineConversion=off
  PWM Blocking1 : Subsystem
  Product : Product
  Simulink-PS Converter : nesl_utility/Simulink-PS Converter  PhysicalDomain=network_engine_domain  SubClassName=ps_input  LeftPortType=input  RightPortType=output  PseudoPeriodic=off  Frequencies=[]  NoiseDistribution=none  NoiseParameters=[]  Unit=1  AffineConversion=off  FilteringAndDerivatives=provide  SimscapeFilterOrder=1  InputFilterTimeConstant=0.001  UdotUserProvided=0
  Simulink-PS Converter2 : nesl_utility/Simulink-PS Converter  PhysicalDomain=network_engine_domain  SubClassName=ps_input  LeftPortType=input  RightPortType=output  PseudoPeriodic=off  Frequencies=[]  NoiseDistribution=none  NoiseParameters=[]  Unit=1  AffineConversion=off  FilteringAndDerivatives=zero  SimscapeFilterOrder=1  InputFilterTimeConstant=0.001  UdotUserProvided=1
  Switch : fl_lib/Electrical/Electrical Elements/Switch  R_closed=0.001*scaling_factor Ohm  G_open=1e-8 1/Ohm  Threshold=0.5  i_specify=off  i_priority=None  i=0 A  i_nominal_specify=off  i_nominal_value=1  i_nominal_unit=A  v_specify=off  v_priority=None  v=0 V  v_nominal_specify=off  v_nominal_value=1  v_nominal_unit=V
  _C1 : fl_lib/Electrical/Electrical Elements/Capacitor  c=C1 F  r=1e-6 Ohm  g=0 1/Ohm  i_specify=off  i_priority=None  i=0 A  i_nominal_specify=off  i_nominal_value=1  i_nominal_unit=A  v_specify=off  v_priority=None  v=0 V  v_nominal_specify=off  v_nominal_value=1  v_nominal_unit=V  vc_specify=off  vc_priority=None  vc=0 V  vc_nominal_specify=off  vc_nominal_value=1  vc_nominal_unit=V
  _L1 : fl_lib/Electrical/Electrical Elements/Inductor  l=L1 H  r=0 Ohm  g=1e-9 1/Ohm  i_specify=off  i_priority=None  i=0 A  i_nominal_specify=off  i_nominal_value=1  i_nominal_unit=A  v_specify=off  v_priority=None  v=0 V  v_nominal_specify=off  v_nominal_value=1  v_nominal_unit=V  i_L_specify=off  i_L_priority=None  i_L=0 A  i_L_nominal_specify=off  i_L_nominal_value=1  i_L_nominal_unit=A
  _R1 : fl_lib/Electrical/Electrical Elements/Resistor  R=R_L1 Ohm  i_specify=off  i_priority=None  i=0 A  i_nominal_specify=off  i_nominal_value=1  i_nominal_unit=A  v_specify=off  v_priority=None  v=0 V  v_nominal_specify=off  v_nominal_value=1  v_nominal_unit=V
  _RC1 : fl_lib/Electrical/Electrical Elements/Resistor  R=R_C1 Ohm  i_specify=off  i_priority=None  i=0 A  i_nominal_specify=off  i_nominal_value=1  i_nominal_unit=A  v_specify=off  v_priority=None  v=0 V  v_nominal_specify=off  v_nominal_value=1  v_nominal_unit=V
  u_cap : fl_lib/Electrical/Electrical Sensors/Voltage Sensor
  u_out : fl_lib/Electrical/Electrical Sensors/Voltage Sensor
  _Ph : PMIOPort  Side=Left
  _N : PMIOPort  Port=2  Side=Left
  _M : PMIOPort  Port=3  Side=Right
  meas : Outport  VectorParamsAs1DForOutWhenUnconnected=off
  wires:
  Bus Selector/2 -> [duty]  "<pwm>"
  Bus Selector/1 -> [connect]  "<connect>"
  [connect] -> Bus Creator2/6  "connection_state"
  ctrl/1 -> Bus Selector/1
  [i_out] -> Bus Creator2/5  "meas_i_out"
  [i_inv] -> Bus Creator2/4  "meas_i_inverter"
  [u_out] -> Bus Creator2/3  "meas_u_out"
  [u_cap] -> Bus Creator2/2  "meas_u_cap"
  Bus Selector/3 -> [enable]  "<enable>"
  [enable] -> Bus Creator2/7  "enabled"
  Bus Creator2/1 -> meas/1
  [u_dc] -> Bus Creator2/1  "meas_u_dc"
  PS-Simulink Converter/1 -> [u_cap]
  PS-Simulink Converter1/1 -> [i_inv]
  PS-Simulink Converter2/1 -> [u_out]
  Product/1 -> Simulink-PS Converter2/1
  Constant/1 -> [u_dc], Gain/1
  [duty] -> Product/1
  Gain/1 -> Product/2
  PS-Simulink Converter3/1 -> [i_out]
  Constant2/1 -> Add1/2
  Add1/1 -> Gain1/1
  Gain3/1 -> PWM Blocking1/1(i_inverter)
  [i_inv] -> Gain3/1
  PWM Blocking1/1(enable_blk) -> Bus Creator2/8, Simulink-PS Converter/1  "block"
  [enable] -> Add1/1
  Gain1/1 -> PWM Blocking1/2(enable)
  connections:
  _R1/RConn1 -- _L1/LConn1
  Current Sensor1/RConn2 -- _L1/RConn1
  _RC1/LConn1 -- Current Sensor/LConn1 -- u_cap/LConn1 -- _R1/LConn1
  DC Voltage Source/RConn1 -- _M/RConn1 -- u_cap/RConn2 -- _C1/RConn1 -- Controlled Voltage Source/RConn2 -- DC Voltage Source1/LConn1
  u_out/LConn1 -- _Ph/RConn1 -- Current Sensor/RConn2
  u_out/RConn2 -- _N/RConn1
  Simulink-PS Converter2/RConn1 -- Controlled Voltage Source/RConn1
  PS-Simulink Converter/LConn1 -- u_cap/RConn1
  PS-Simulink Converter1/LConn1 -- Current Sensor1/RConn1
  PS-Simulink Converter2/LConn1 -- u_out/RConn1
  PS-Simulink Converter3/LConn1 -- Current Sensor/RConn1
  _RC1/RConn1 -- _C1/LConn1
  Diode1/RConn1 -- Current Sensor1/LConn1 -- Switch/RConn2 -- Diode/LConn1
  Controlled Voltage Source/LConn1 -- Switch/LConn1
  Simulink-PS Converter/RConn1 -- Switch/RConn1
  Current Sensor3/LConn1 -- DC Voltage Source1/RConn1
  Current Sensor3/RConn2 -- Diode1/LConn1
  PS-Simulink Converter4/LConn1 -- Current Sensor2/RConn1
  Current Sensor2/RConn2 -- Diode/RConn1
  PS-Simulink Converter5/LConn1 -- Current Sensor3/RConn1
  Current Sensor2/LConn1 -- DC Voltage Source/LConn1

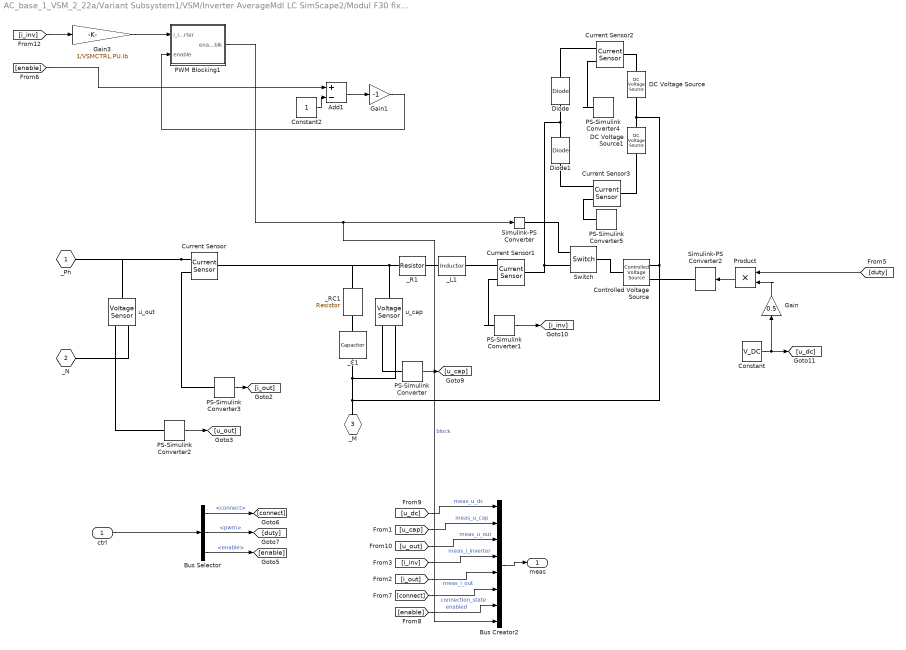
== system AC_base_1_VSM_2_22a/Variant Subsystem1/VSM/Inverter AverageMdl LC SimScape2/Modul F30 fixed DC voltage Average SimScape/simscape_bridgefilter_aca2 ==
  ctrl : Inport
  Add1 : Sum  Inputs=+-
  Bus Creator2 : BusCreator  Inputs=8
  Bus Selector : BusSelector  OutputSignals=connect,pwm,enable
  Constant : Constant  Value=V_DC
  Constant2 : Constant
  Controlled Voltage Source : fl_lib/Electrical/Electrical Sources/Controlled Voltage Source
  Current Sensor{,1..3} (4 alike) : fl_lib/Electrical/Electrical Sensors/Current Sensor
  DC Voltage Source : fl_lib/Electrical/Electrical Sources/DC Voltage Source  v0=V_DC/2 V
  DC Voltage Source1 : fl_lib/Electrical/Electrical Sources/DC Voltage Source  v0=V_DC/2 V
  Diode : fl_lib/Electrical/Electrical Elements/Diode  Vf=0.6 V  Ron=0.001*scaling_factor Ohm  Goff=1e-8 1/Ohm  i_specify=off  i_priority=None  i=0 A  i_nominal_specify=off  i_nominal_value=1  i_nominal_unit=A  v_specify=off  v_priority=None  v=0 V  v_nominal_specify=off  v_nominal_value=1  v_nominal_unit=V
  Diode1 : fl_lib/Electrical/Electrical Elements/Diode  Vf=0.6 V  Ron=0.001*scaling_factor Ohm  Goff=1e-8 1/Ohm  i_specify=off  i_priority=None  i=0 A  i_nominal_specify=off  i_nominal_value=1  i_nominal_unit=A  v_specify=off  v_priority=None  v=0 V  v_nominal_specify=off  v_nominal_value=1  v_nominal_unit=V
  Gain : Gain  Gain=0.5
  Gain1 : Gain  Gain=-1
  Gain3 : Gain  Gain=1/VSMCTRL.PU.Ib
  PS-Simulink Converter{,1..5} (6 alike) : nesl_utility/PS-Simulink Converter  PhysicalDomain=network_engine_domain  SubClassName=ps_output  LeftPortType=input  RightPortType=output  PseudoPeriodic=off  Frequencies=[]  VectorFormat=1-D array  Unit=1  AffineConversion=off
  PWM Blocking1 : Subsystem
  Product : Product
  Simulink-PS Converter : nesl_utility/Simulink-PS Converter  PhysicalDomain=network_engine_domain  SubClassName=ps_input  LeftPortType=input  RightPortType=output  PseudoPeriodic=off  Frequencies=[]  NoiseDistribution=none  NoiseParameters=[]  Unit=1  AffineConversion=off  FilteringAndDerivatives=provide  SimscapeFilterOrder=1  InputFilterTimeConstant=0.001  UdotUserProvided=0
  Simulink-PS Converter2 : nesl_utility/Simulink-PS Converter  PhysicalDomain=network_engine_domain  SubClassName=ps_input  LeftPortType=input  RightPortType=output  PseudoPeriodic=off  Frequencies=[]  NoiseDistribution=none  NoiseParameters=[]  Unit=1  AffineConversion=off  FilteringAndDerivatives=zero  SimscapeFilterOrder=1  InputFilterTimeConstant=0.001  UdotUserProvided=1
  Switch : fl_lib/Electrical/Electrical Elements/Switch  R_closed=0.001*scaling_factor Ohm  G_open=1e-8 1/Ohm  Threshold=0.5  i_specify=off  i_priority=None  i=0 A  i_nominal_specify=off  i_nominal_value=1  i_nominal_unit=A  v_specify=off  v_priority=None  v=0 V  v_nominal_specify=off  v_nominal_value=1  v_nominal_unit=V
  _C1 : fl_lib/Electrical/Electrical Elements/Capacitor  c=C1 F  r=1e-6 Ohm  g=0 1/Ohm  i_specify=off  i_priority=None  i=0 A  i_nominal_specify=off  i_nominal_value=1  i_nominal_unit=A  v_specify=off  v_priority=None  v=0 V  v_nominal_specify=off  v_nominal_value=1  v_nominal_unit=V  vc_specify=off  vc_priority=None  vc=0 V  vc_nominal_specify=off  vc_nominal_value=1  vc_nominal_unit=V
  _L1 : fl_lib/Electrical/Electrical Elements/Inductor  l=L1 H  r=0 Ohm  g=1e-9 1/Ohm  i_specify=off  i_priority=None  i=0 A  i_nominal_specify=off  i_nominal_value=1  i_nominal_unit=A  v_specify=off  v_priority=None  v=0 V  v_nominal_specify=off  v_nominal_value=1  v_nominal_unit=V  i_L_specify=off  i_L_priority=None  i_L=0 A  i_L_nominal_specify=off  i_L_nominal_value=1  i_L_nominal_unit=A
  _R1 : fl_lib/Electrical/Electrical Elements/Resistor  R=R_L1 Ohm  i_specify=off  i_priority=None  i=0 A  i_nominal_specify=off  i_nominal_value=1  i_nominal_unit=A  v_specify=off  v_priority=None  v=0 V  v_nominal_specify=off  v_nominal_value=1  v_nominal_unit=V
  _RC1 : fl_lib/Electrical/Electrical Elements/Resistor  R=R_C1 Ohm  i_specify=off  i_priority=None  i=0 A  i_nominal_specify=off  i_nominal_value=1  i_nominal_unit=A  v_specify=off  v_priority=None  v=0 V  v_nominal_specify=off  v_nominal_value=1  v_nominal_unit=V
  u_cap : fl_lib/Electrical/Electrical Sensors/Voltage Sensor
  u_out : fl_lib/Electrical/Electrical Sensors/Voltage Sensor
  _Ph : PMIOPort  Side=Left
  _N : PMIOPort  Port=2  Side=Left
  _M : PMIOPort  Port=3  Side=Right
  meas : Outport  VectorParamsAs1DForOutWhenUnconnected=off
  wires:
  Gain1/1 -> PWM Blocking1/2(enable)
  [enable] -> Add1/1
  PWM Blocking1/1(enable_blk) -> Simulink-PS Converter/1, Bus Creator2/8  "block"
  [i_inv] -> Gain3/1
  Gain3/1 -> PWM Blocking1/1(i_inverter)
  Add1/1 -> Gain1/1
  Constant2/1 -> Add1/2
  PS-Simulink Converter3/1 -> [i_out]
  Gain/1 -> Product/2
  [duty] -> Product/1
  Constant/1 -> Gain/1, [u_dc]
  Product/1 -> Simulink-PS Converter2/1
  PS-Simulink Converter2/1 -> [u_out]
  PS-Simulink Converter1/1 -> [i_inv]
  PS-Simulink Converter/1 -> [u_cap]
  [u_dc] -> Bus Creator2/1  "meas_u_dc"
  Bus Creator2/1 -> meas/1
  [enable] -> Bus Creator2/7  "enabled"
  Bus Selector/3 -> [enable]  "<enable>"
  [u_cap] -> Bus Creator2/2  "meas_u_cap"
  [u_out] -> Bus Creator2/3  "meas_u_out"
  [i_inv] -> Bus Creator2/4  "meas_i_inverter"
  [i_out] -> Bus Creator2/5  "meas_i_out"
  ctrl/1 -> Bus Selector/1
  [connect] -> Bus Creator2/6  "connection_state"
  Bus Selector/1 -> [connect]  "<connect>"
  Bus Selector/2 -> [duty]  "<pwm>"
  connections:
  Current Sensor2/LConn1 -- DC Voltage Source/LConn1
  PS-Simulink Converter5/LConn1 -- Current Sensor3/RConn1
  Current Sensor2/RConn2 -- Diode/RConn1
  PS-Simulink Converter4/LConn1 -- Current Sensor2/RConn1
  Current Sensor3/RConn2 -- Diode1/LConn1
  Current Sensor3/LConn1 -- DC Voltage Source1/RConn1
  Simulink-PS Converter/RConn1 -- Switch/RConn1
  Controlled Voltage Source/LConn1 -- Switch/LConn1
  Diode/LConn1 -- Switch/RConn2 -- Current Sensor1/LConn1 -- Diode1/RConn1
  _RC1/RConn1 -- _C1/LConn1
  PS-Simulink Converter3/LConn1 -- Current Sensor/RConn1
  PS-Simulink Converter2/LConn1 -- u_out/RConn1
  PS-Simulink Converter1/LConn1 -- Current Sensor1/RConn1
  PS-Simulink Converter/LConn1 -- u_cap/RConn1
  Simulink-PS Converter2/RConn1 -- Controlled Voltage Source/RConn1
  u_out/RConn2 -- _N/RConn1
  Current Sensor/RConn2 -- _Ph/RConn1 -- u_out/LConn1
  DC Voltage Source1/LConn1 -- Controlled Voltage Source/RConn2 -- _C1/RConn1 -- u_cap/RConn2 -- _M/RConn1 -- DC Voltage Source/RConn1
  _R1/LConn1 -- u_cap/LConn1 -- Current Sensor/LConn1 -- _RC1/LConn1
  Current Sensor1/RConn2 -- _L1/RConn1
  _R1/RConn1 -- _L1/LConn1

== system AC_base_1_VSM_2_22a/Variant Subsystem1/VSM/VSM1/VSM/BUS_GENERATION ==
  MANAGE : Inport
  CONTROL : Inport  Port=2
  Bus Creator1 : BusCreator  Inputs=4
  Bus Selector2 : BusSelector  OutputSignals=PWM
  Bus Selector3 : BusSelector  OutputSignals=ENABLED,CONNECT
  Bus Selector4 : BusSelector  OutputSignals=CONNECTED,ENABLED
  Bus Creator6 : BusCreator  Inputs=2  OutDataTypeStr=Bus: FeedbackACBus
  Data Type Conversion{,1..3} (4 alike) : DataTypeConversion  SaturateOnIntegerOverflow=off  RndMeth=Floor
  Signal Specification1 : SignalSpecification
  additional data1 : Constant  Value=0
  ctrl : Outport  VectorParamsAs1DForOutWhenUnconnected=off
  feedback : Outport  Port=2  VectorParamsAs1DForOutWhenUnconnected=off
  wires:
  Bus Selector2/1 -> Signal Specification1/1  "<PWM>"
  Bus Selector4/1 -> Data Type Conversion3/1  "<CONNECTED>"
  Bus Selector4/2 -> Data Type Conversion2/1  "<ENABLED>"
  CONTROL/1 -> Bus Selector2/1
  Data Type Conversion2/1 -> Bus Creator6/2  "enabled"
  Signal Specification1/1 -> Bus Creator1/1  "pwm"
  MANAGE/1 -> Bus Selector3/1, Bus Selector4/1
  Bus Creator1/1 -> ctrl/1
  Bus Creator6/1 -> feedback/1
  Bus Selector3/1 -> Data Type Conversion/1  "<ENABLED>"
  Data Type Conversion/1 -> Bus Creator1/2  "enable"
  Data Type Conversion1/1 -> Bus Creator1/3  "connect"
  additional data1/1 -> Bus Creator1/4  "source_id"
  Bus Selector3/2 -> Data Type Conversion1/1  "<CONNECT>"
  Data Type Conversion3/1 -> Bus Creator6/1  "connected"

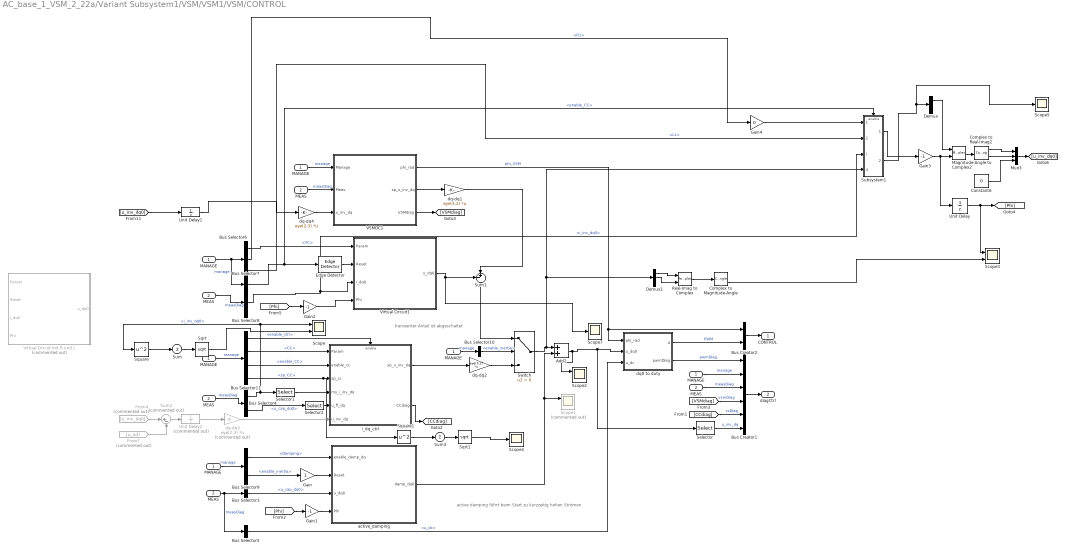
== system AC_base_1_VSM_2_22a/Variant Subsystem1/VSM/VSM1/VSM/CONTROL ==
  note: transienter Anteil ist abgeschaltet
  note: active damping führt beim Start zu kurzzeitig hohen Strömen
  MANAGE : Inport
  MEAS : Inport  Port=2
  "  MANAGE " : InportShadow
  "  MEAS " : InportShadow  Port=2
  "  MEAS  " : InportShadow  Port=2
  " MANAGE" : InportShadow
  " MEAS" : InportShadow  Port=2
  Add2 : Sum
  Bus Creator1 : BusCreator  Inputs=6
  Bus Creator2 : BusCreator  Inputs=2
  Bus Selector10 : BusSelector  OutputSignals=enable_VSM.enable_inertia
  Bus Selector11 : BusSelector  OutputSignals=enable_VSM.enable_ctrl,Param.CC,enable_CC,sp_CC
  Bus Selector3 : BusSelector  OutputSignals=u_cap.u_cap_dq0
  Bus Selector4 : BusSelector  OutputSignals=i_inv.i_inv_dq0,u_cap.u_cap_dq0
  Bus Selector5 : BusSelector  OutputSignals=u_dc
  Bus Selector6 : BusSelector  OutputSignals=Param.VC,Param.VC.R1,Param.VC.L1
  Bus Selector7 : BusSelector  OutputSignals=enable_CC
  Bus Selector8 : BusSelector  OutputSignals=i_inv.i_inv_dq0
  Bus Selector9 : BusSelector  OutputSignals=Param.Damping,enable_VSM.enable_inertia
  Complex to Magnitude-Angle : ComplexToMagnitudeAngle
  Complex to Real-Imag2 : ComplexToRealImag
  Constant6 : Constant  Value=0
  Demux : Demux  Outputs=2
  Demux1 : Demux  Outputs=3
  Edge Detector : spsEdgeDetectorLib/Edge Detector  model=Falling  ic=0  Ts=0
  From4 : From  Commented=on  GotoTag=u_inv_dq0
  From7 : From  Commented=on  GotoTag=u_ad
  Gain : Gain
  Gain1 : Gain  Gain=-1
  Gain2 : Gain  Gain=-1
  Gain3 : Gain  Gain=-1
  Gain4 : Gain  Gain=0
  "MANAGE  " : InportShadow
  "MANAGE   " : InportShadow
  "MANAGE    " : InportShadow
  "MEAS " : InportShadow  Port=2
  Magnitude-Angle to Complex2 : MagnitudeAngleToComplex
  Mux3 : Mux  Inputs=3
  Real-Imag to Complex : RealImagToComplex
  Scope : Scope  NumInputPorts=2
  Scope1 : Scope  Commented=on  NumInputPorts=2
  Scope2 : Scope  NumInputPorts=2
  Scope3 : Scope  NumInputPorts=2
  Scope4 : Scope
  Scope5 : Scope
  Scope7 : Scope  NumInputPorts=3
  Selector : Selector  InputPortWidth=3  IndexOptions=Index vector (dialog)  Indices=[1 2]  OutputSizes=1
  Selector1 : Selector  InputPortWidth=3  IndexOptions=Index vector (dialog)  Indices=[1 2]  OutputSizes=1
  Selector2 : Selector  InputPortWidth=3  IndexOptions=Index vector (dialog)  Indices=[1 2]  OutputSizes=1
  Sqrt : Sqrt
  Sqrt1 : Sqrt
  Square : Math  Operator=square
  Square1 : Math  Operator=square
  Subsystem1 : Subsystem
  Sum : Sum  Inputs=+
  Sum1 : Sum  Inputs=-+|
  Sum2 : Sum  Commented=on  Inputs=|+-
  Sum3 : Sum  Inputs=+
  Switch : Switch  Criteria=u2 > Threshold  SaturateOnIntegerOverflow=off  InputSameDT=off
  Unit Delay : UnitDelay  SampleTime=-1  HasFrameUpgradeWarning=on
  Unit Delay1 : UnitDelay  SampleTime=ControlSampleTime  HasFrameUpgradeWarning=on
  Unit Delay2 : UnitDelay  Commented=on  SampleTime=ControlSampleTime  HasFrameUpgradeWarning=on
  VSMOC1 : Subsystem  mask(VSM mit OC){VSM=Ctrl.VSM}
      mask prompts: VSM "VSM Parameter"
      mask help:
      | VSM(.Ta, .kpf, .kdf, .f0, .ku, .Tu)
      |
      | Parameter nicht auf der Maske:
      | ControlSampleTime
  Virtual Circuit mit R und L : Subsystem  Commented=on  AncestorBlock=ControLibrary/Virtual Circuit
  Virtual Circuit1 : Subsystem  AncestorBlock=ControLibrary/Virtual Circuit
  active_damping : Subsystem  mask(Lead Lag){OmLead=Ctrl.VTFF.OmLead, OmLag=Ctrl.VTFF.OmLag}
      mask prompts: OmLead "Omega Lead"; OmLag "Omega Lag"
  dq-dq1 : Gain  Gain=eye(3,2)  Multiplication=Matrix(K*u)
  dq-dq2 : Gain  Gain=eye(3,2)  Multiplication=Matrix(K*u)
  dq-dq3 : Gain  Commented=on  Gain=eye(2,3)  Multiplication=Matrix(K*u)
  dq-dq4 : Gain  Gain=eye(2,3)  Multiplication=Matrix(K*u)
  dq0 to duty : Subsystem
  i_dq_ctrl : Subsystem  mask(PI DQ Stromregler){Kp=Ctrl.CC.kp*0+0.28*2.5/2, Ki=Ctrl.CC.ki*0+28*20/2, L_inv=Ctrl.CC.xff, Kff=Ctrl.CC.Kff}
      mask prompts: Kp "P-Anteil:"; Ki "I-Anteil:"; L_inv "Induktivität [pu]:"; Kff "Vorsteuerung"
      mask help:
      | - in pu Einheiten
      | - 2-phasige DQ Regelung
      | - Entkopplung der d- und q-Achse
      | - Vorsteuerung der Kondensatorspannung
      | - Aktive Dämpfung der LC-Filter Resonanz
      | - Aktive Dämpfung der Zwischenkreis Spannung
  CONTROL : Outport  VectorParamsAs1DForOutWhenUnconnected=off
  diagCtrl : Outport  Port=2  VectorParamsAs1DForOutWhenUnconnected=off
  wires:
  Square1/1 -> Sum3/1
  Sum3/1 -> Sqrt1/1
  Sqrt1/1 -> Scope4/1
  Complex to Magnitude-Angle/2 -> Scope3/2
  Real-Imag to Complex/1 -> Complex to Magnitude-Angle/1
  Demux1/1 -> Real-Imag to Complex/1
  Demux1/2 -> Real-Imag to Complex/2
  Unit Delay/1 -> [Phi], Scope3/1
  Sqrt/1 -> Scope/2
  Sum/1 -> Sqrt/1
  Square/1 -> Sum/1
  Gain4/1 -> Subsystem1/1(<R1>)
  Edge Detector/1 -> Virtual Circuit1/2(Reset)
  Demux/1 -> Magnitude-Angle to Complex2/1
  active_damping/1(damp_dq0) -> Add2/2, Scope1/1
  Complex to Real-Imag2/2 -> Mux3/2
  Complex to Real-Imag2/1 -> Mux3/1
  Switch/1 -> Add2/1, Subsystem1/4(U_i), Demux1/1
  i_dq_ctrl/1(sp_u_inv_dq) -> dq-dq2/1
  Gain3/1 -> Magnitude-Angle to Complex2/2, Unit Delay/1
  dq-dq4/1 -> VSMOC1/3(u_inv_dq)
  Subsystem1/2(U_v) -> Demux/1, Scope5/1
  Subsystem1/1(phi_vsm) -> Gain3/1
  dq-dq1/1 -> Sum1/2
  Mux3/1 -> [u_inv_dq0]
  Constant6/1 -> Mux3/3
  Magnitude-Angle to Complex2/1 -> Complex to Real-Imag2/1
  [u_inv_dq0] -> Unit Delay1/1
  Bus Selector6/3 -> Subsystem1/2(<L1>)  "<L1>"
  Bus Selector6/2 -> Gain4/1  "<R1>"
  Virtual Circuit1/1(" u_dq0") -> Sum1/1, Scope7/2
  Bus Selector7/1 -> Subsystem1/Enable, Edge Detector/1  "<enable_CC>"
  Bus Selector8/1 -> Subsystem1/3(I), Virtual Circuit1/3(i_dq0)  "<i_inv_dq0>"
  Bus Selector11/4 -> i_dq_ctrl/3(sp_cc), Square1/1  "<sp_CC>"
  Selector1/1 -> i_dq_ctrl/4(ms_i_inv_dq)
  Bus Selector4/2 -> Selector2/1  "<u_cap_dq0>"
  Bus Selector11/3 -> i_dq_ctrl/2(enable_cc)  "<enable_CC>"
  Gain2/1 -> Virtual Circuit1/4(Phi)
  [Phi] -> Gain2/1
  From7/1 -> Sum2/2
  From4/1 -> Sum2/1
  Sum2/1 -> Unit Delay2/1
  Gain1/1 -> active_damping/4(Phi)
  Gain/1 -> active_damping/2(Reset)
  Bus Selector9/2 -> Gain/1  "<enable_inertia>"
  Bus Selector3/1 -> active_damping/3(u_dq0)  "<u_cap_dq0>"
  Unit Delay2/1 -> dq-dq3/1
  VSMOC1/1(phi_rad) -> dq0 to duty/1(phi_rad), Bus Creator2/1  "phi_VSM"
  Bus Selector6/1 -> Virtual Circuit1/1(Param)  "<VC>"
  "MANAGE   "/1 -> Bus Selector6/1, Bus Selector7/1  "manage"
  "  MEAS  "/1 -> Bus Selector8/1  "measDiag"
  Selector/1 -> Bus Creator1/6  "u_inv_dq"
  VSMOC1/2(sp_u_inv_dq) -> dq-dq1/1
  Bus Selector5/1 -> dq0 to duty/3(u_dc)  "<u_dc>"
  [CCdiag] -> Bus Creator1/5  "ccDiag"
  "MANAGE  "/1 -> Bus Selector10/1  "manage"
  Bus Selector10/1 -> Switch/2  "<enable_inertia>"
  i_dq_ctrl/2(CCdiag) -> [CCdiag]
  Bus Selector4/1 -> Selector1/1, Scope/1, Square/1  "<i_inv_dq0>"
  "MEAS "/1 -> Bus Selector4/1  "measDiag"
  "MANAGE    "/1 -> Bus Selector11/1  "manage"
  Bus Selector11/1 -> i_dq_ctrl/Enable  "<enable_ctrl>"
  Selector2/1 -> i_dq_ctrl/5(u_ff_dq)
  Bus Selector11/2 -> i_dq_ctrl/1(Param)  "<CC>"
  dq-dq3/1 -> i_dq_ctrl/6(u_inv_dq)
  Add2/1 -> dq0 to duty/2(u_dq0), Selector/1, Scope2/1
  MEAS/1 -> VSMOC1/2(Meas)  "measDiag"
  Bus Creator2/1 -> CONTROL/1
  " MEAS"/1 -> Bus Selector5/1, Bus Selector3/1  "measDiag"
  "  MANAGE "/1 -> Bus Creator1/2  "manage"
  Bus Creator1/1 -> diagCtrl/1
  Bus Selector9/1 -> active_damping/1(enable_damp_dq)  "<Damping>"
  " MANAGE"/1 -> Bus Selector9/1  "manage"
  dq0 to duty/2(pwmDiag) -> Bus Creator1/1  "pwmDiag"
  MANAGE/1 -> VSMOC1/1(Manage)  "manage"
  dq0 to duty/1(d) -> Bus Creator2/2  "PWM"
  VSMOC1/3(VSMdiag) -> [VSMdiag]
  "  MEAS "/1 -> Bus Creator1/3  "measDiag"
  [VSMdiag] -> Bus Creator1/4  "vsmDiag"
  Sum1/1 -> Switch/1
  dq-dq2/1 -> Switch/3
  Unit Delay1/1 -> dq-dq4/1
  [Phi] -> Gain1/1
